simulink model "d_ChaineAir"  (R2024b)
settings: Solver=VariableStepAuto  StartTime=0.0  StopTime=10.0  RelTol=1e-3
values from neighbouring files (symbols this model uses):
  gam = 1.4    [InitISM_AII.m]
  Mim0 = 0+0.001    (= 0.001)    [InitISM_AII.m]
  nv_remp = [0.090 0.110 0.120 0.110 0.130 0.150 0.135 0.155 0.140 0.145 0.140 0.135 0.120 0.120 ... (first row only)    [InitISM_AII.m]
  Pamb = 101300    [InitISM_AII.m]
  PRcrit = ((gam+1)/2)^(gam/(1-gam))    (= 0.528281787717)    [InitISM_AII.m]
  Rair = 287.0    (= 287)    [InitISM_AII.m]
  Tamb = 300    [InitISM_AII.m]
  Vcyl = 1998e-6/4    (= 0.0004995)    [InitISM_AII.m]
undefined symbols (not defined in the file or in its folder): AirMotTest, AirPapTest, AirPressureTest, AirTimeTest, P0, PcolPapTest, RegimeTest, SectionPapTest, TempsPapTest, TempsTest
settings Model: Creator=a030141  LastModifiedBy=ramse
settings DebuggingCC: UnderspecifiedInitializationDetection=Classic  MergeDetectMultiDrivingBlocksExec=none
settings ModelReferenceCC: PropagateSignalLabelsOutOfModel=off

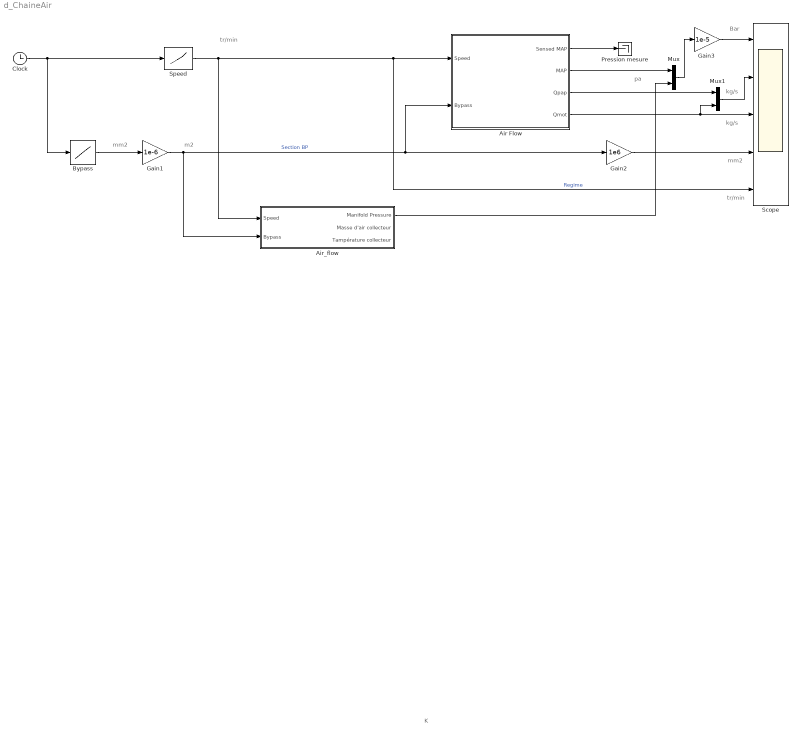
== system d_ChaineAir ==
  note: pa
  note: Bar
  note: tr/min
  note: tr/min
  note: m2
  note: mm2
  note: mm2
  note: kg/s
  note: kg/s
  note: K
  Air Flow : Subsystem
  Air_flow : Subsystem
  Bypass : Lookup  InputValues=TempsPapTest  Table=SectionPapTest.*PcolPapTest
  Clock : Clock
  Gain1 : Gain  Gain=1e-6  SaturateOnIntegerOverflow=on  OutDataTypeStr=Inherit: Same as input  ParamDataTypeStr=Inherit: Same as input
  Gain2 : Gain  Gain=1e6  SaturateOnIntegerOverflow=on  OutDataTypeStr=Inherit: Same as input  ParamDataTypeStr=Inherit: Same as input
  Gain3 : Gain  Gain=1e-5  SaturateOnIntegerOverflow=on  OutDataTypeStr=Inherit: Same as input  ParamDataTypeStr=Inherit: Same as input
  Mux : Mux  Inputs=2
  Mux1 : Mux  Inputs=2
  Pression mesure : Terminator
  Scope : Scope  NumInputPorts=5
  Speed : Lookup  InputValues=TempsTest  Table=RegimeTest
  wires:
  Clock/1 -> Speed/1, Bypass/1
  Bypass/1 -> Gain1/1
  Air Flow/2(MAP) -> Mux/1
  Mux/1 -> Gain3/1
  Gain3/1 -> Scope/1
  Air Flow/4(Qmot) -> Scope/3, Mux1/2
  Gain2/1 -> Scope/4
  Mux1/1 -> Scope/2
  Air Flow/1(Sensed MAP) -> Pression mesure/1
  Gain1/1 -> Air_flow/2(Bypass), Gain2/1, Air Flow/2(Bypass)  "Section BP"
  Air Flow/3(Qpap) -> Mux1/1
  Speed/1 -> Air_flow/1(Speed), Scope/5, Air Flow/1(Speed)  "Regime"
  Air_flow/1(Manifold Pressure) -> Mux/2

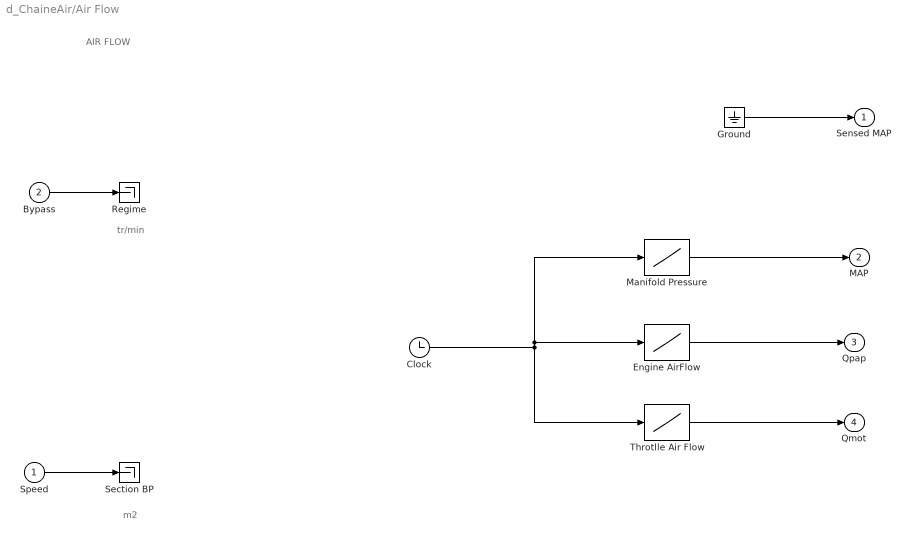
== system d_ChaineAir/Air Flow ==
  note: AIR FLOW
  note: m2
  note: tr/min
  Speed : Inport
  Bypass : Inport  Port=2
  Clock : Clock
  Engine AirFlow : Lookup  InputValues=AirTimeTest  Table=AirMotTest
  Ground : Ground
  Manifold Pressure : Lookup  InputValues=AirTimeTest  Table=AirPressureTest
  Regime : Terminator
  Section BP : Terminator
  Throtlle Air Flow : Lookup  InputValues=AirTimeTest  Table=AirPapTest
  Sensed MAP : Outport
  MAP : Outport  Port=2
  Qpap : Outport  Port=3
  Qmot : Outport  Port=4
  wires:
  Bypass/1 -> Regime/1
  Speed/1 -> Section BP/1
  Ground/1 -> Sensed MAP/1
  Clock/1 -> Manifold Pressure/1, Engine AirFlow/1, Throtlle Air Flow/1
  Manifold Pressure/1 -> MAP/1
  Throtlle Air Flow/1 -> Qmot/1
  Engine AirFlow/1 -> Qpap/1

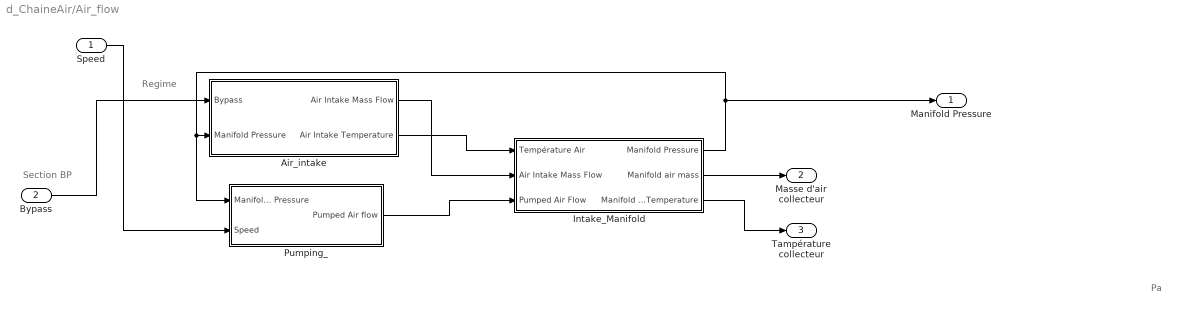
== system d_ChaineAir/Air_flow ==
  note: Section BP
  note: Regime
  note: Pa
  Speed : Inport
  Bypass : Inport  Port=2
  Air_intake : Subsystem
  Intake_Manifold : Subsystem
  Pumping_ : Subsystem
  Manifold Pressure : Outport
  Masse d'air collecteur : Outport  Port=2
  Tampérature collecteur : Outport  Port=3
  wires:
  Speed/1 -> Pumping_/2(Speed)
  Intake_Manifold/2(Manifold air mass) -> Masse d'air collecteur/1
  Intake_Manifold/1(Manifold Pressure) -> Manifold Pressure/1, Pumping_/1(Manifold Pressure), Air_intake/2(Manifold Pressure)
  Bypass/1 -> Air_intake/1(Bypass)
  Intake_Manifold/3(Manifold Temperature) -> Tampérature collecteur/1
  Air_intake/2(Air Intake Temperature) -> Intake_Manifold/1(Température Air)
  Air_intake/1(Air Intake Mass Flow) -> Intake_Manifold/2(Air Intake Mass Flow)
  Pumping_/1(Pumped Air flow) -> Intake_Manifold/3(Pumped Air Flow)

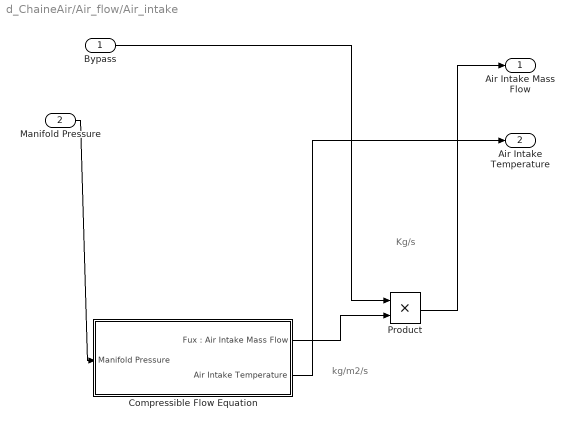
== system d_ChaineAir/Air_flow/Air_intake ==
  note: Kg/s
  note: kg/m2/s
  Bypass : Inport
  Manifold Pressure : Inport  Port=2
  Compressible Flow Equation : Subsystem
  Product : Product
  Air Intake Mass Flow : Outport
  Air Intake Temperature : Outport  Port=2
  wires:
  Compressible Flow Equation/2(Air Intake Temperature) -> Air Intake Temperature/1
  Compressible Flow Equation/1("Fux : Air Intake Mass Flow") -> Product/2
  Manifold Pressure/1 -> Compressible Flow Equation/1(Manifold Pressure)
  Product/1 -> Air Intake Mass Flow/1
  Bypass/1 -> Product/1

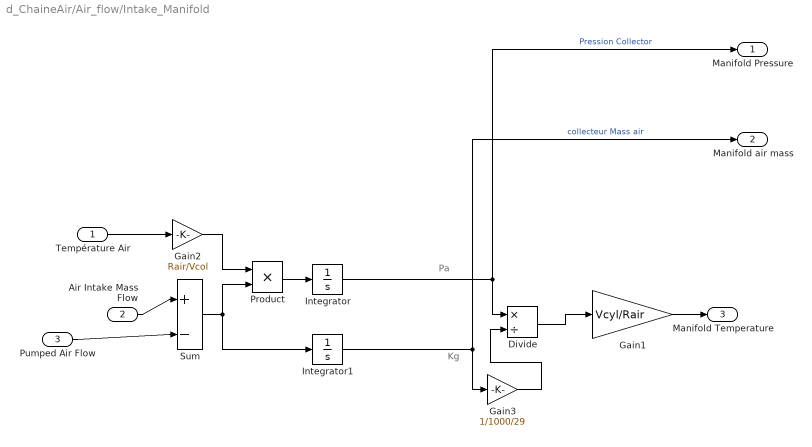
== system d_ChaineAir/Air_flow/Intake_Manifold ==
  note: Kg
  note: Pa
  Température Air : Inport
  Air Intake Mass Flow : Inport  Port=2
  Pumped Air Flow : Inport  Port=3
  Divide : Product  Inputs=*/
  Gain1 : Gain  Gain=Vcyl/Rair
  Gain2 : Gain  Gain=Rair/Vcol
  Gain3 : Gain  Gain=1/1000/29
  Integrator : Integrator  InitialCondition=P0
  Integrator1 : Integrator  InitialCondition=Mim0
  Product : Product
  Sum : Sum  Inputs=|+-
  Manifold Pressure : Outport
  Manifold air mass : Outport  Port=2
  Manifold Temperature : Outport  Port=3
  wires:
  Sum/1 -> Integrator1/1, Product/2
  Gain2/1 -> Product/1
  Product/1 -> Integrator/1
  Gain1/1 -> Manifold Temperature/1
  Integrator/1 -> Manifold Pressure/1, Divide/1  "Pression Collector"
  Integrator1/1 -> Manifold air mass/1, Gain3/1  "collecteur Mass air"
  Gain3/1 -> Divide/2
  Divide/1 -> Gain1/1
  Air Intake Mass Flow/1 -> Sum/1
  Température Air/1 -> Gain2/1
  Pumped Air Flow/1 -> Sum/2

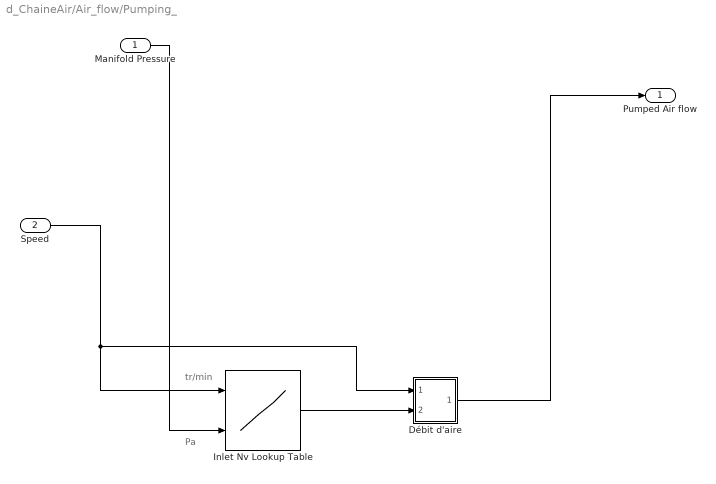
== system d_ChaineAir/Air_flow/Pumping_ ==
  note: Pa
  note: tr/min
  Manifold Pressure : Inport
  Speed : Inport  Port=2
  Débit d'aire : Subsystem
  Inlet Nv Lookup Table : Lookup2D  RowIndex=Ne_remp  ColumnIndex=Pcol_remp  Table=nv_remp
  Pumped Air flow : Outport
  wires:
  Inlet Nv Lookup Table/1 -> Débit d'aire/2(In2)
  Speed/1 -> Inlet Nv Lookup Table/1, Débit d'aire/1(In1)
  Manifold Pressure/1 -> Inlet Nv Lookup Table/2
  Débit d'aire/1(Out1) -> Pumped Air flow/1

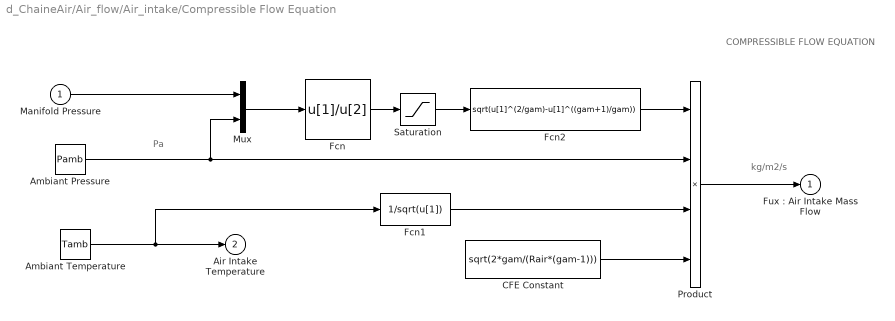
== system d_ChaineAir/Air_flow/Air_intake/Compressible Flow Equation ==
  note: COMPRESSIBLE FLOW EQUATION
  note: Pa
  note: kg/m2/s
  Manifold Pressure : Inport
  Ambiant Pressure : Constant  Value=Pamb
  Ambiant Temperature : Constant  Value=Tamb
  "CFE Constant " : Constant  Value=sqrt(2*gam/(Rair*(gam-1)))
  Fcn : Fcn  Expr=u[1]/u[2]
  Fcn1 : Fcn  Expr=1/sqrt(u[1])
  Fcn2 : Fcn  Expr=sqrt(u[1]^(2/gam)-u[1]^((gam+1)/gam))
  Mux : Mux  Inputs=2
  Product : Product  Inputs=4  InputSameDT=on  SaturateOnIntegerOverflow=on  OutDataTypeStr=Inherit: Same as first input
  Saturation : Saturate  UpperLimit=1  LowerLimit=PRcrit
  "Fux : Air Intake Mass Flow" : Outport
  Air Intake Temperature : Outport  Port=2
  wires:
  Ambiant Pressure/1 -> Product/2, Mux/2
  Product/1 -> "Fux : Air Intake Mass Flow"/1
  "CFE Constant "/1 -> Product/4
  Fcn2/1 -> Product/1
  Saturation/1 -> Fcn2/1
  Fcn1/1 -> Product/3
  Fcn/1 -> Saturation/1
  Mux/1 -> Fcn/1
  Manifold Pressure/1 -> Mux/1
  Ambiant Temperature/1 -> Fcn1/1, Air Intake Temperature/1

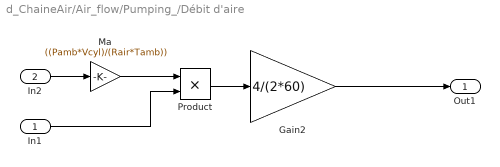
== system d_ChaineAir/Air_flow/Pumping_/Débit d'aire ==
  In1 : Inport
  In2 : Inport  Port=2
  Gain2 : Gain  Gain=4/(2*60)
  Ma : Gain  Gain=((Pamb*Vcyl)/(Rair*Tamb))
  Product : Product
  Out1 : Outport
  wires:
  Ma/1 -> Product/1
  Gain2/1 -> Out1/1
  Product/1 -> Gain2/1
  In1/1 -> Product/2
  In2/1 -> Ma/1
